simulink model "obs_based_state_xfer"  (Simulink 8.6)
settings: Solver=ode45  StartTime=0.0  StopTime=10.0  RelTol=1e-3
settings Model: Creator=Thomas Chmielewski  LastModifiedBy=DR_C
settings OptimizationCC: InitFltsAndDblsToZero=on
settings DebuggingCC: SaveWithParameterizedLinksMsg=none  SignalResolutionControl=TryResolveAllWithWarning  SolverPrmCheckMsg=none  MultiTaskDSMMsg=warning  MultiTaskCondExecSysMsg=none  FcnCallInpInsideContextMsg=UseLocalSettings  StrictBusMsg=None
settings HardwareCC: TargetUnknown=on
settings GRTTargetCC: TargetFcnLib=ansi_tfl_tmw.mat  CompOptLevelCompliant=off  GeneratePreprocessorConditionals=Use local settings

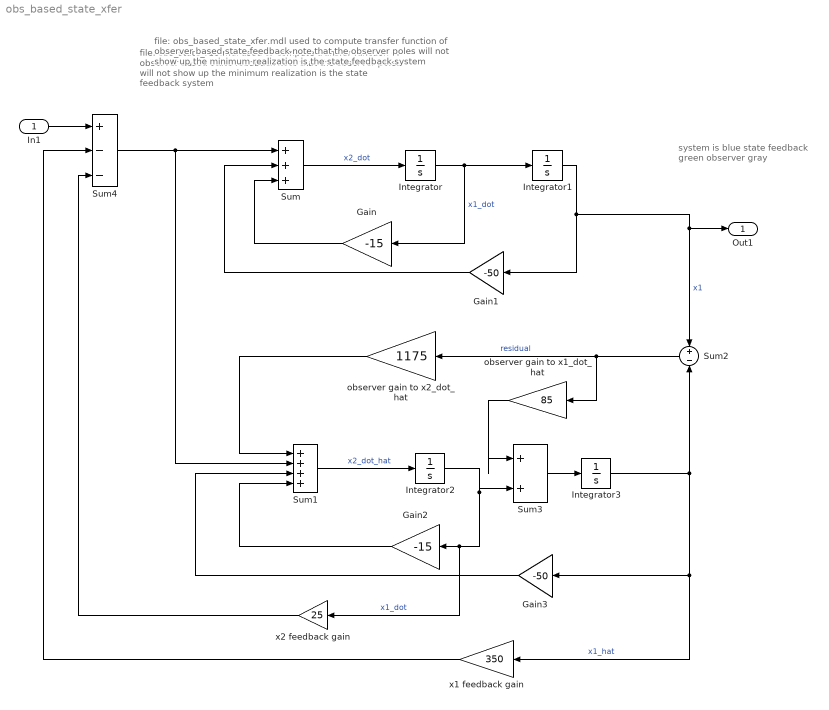
== system obs_based_state_xfer ==
  note: system is blue
      | state feedback green
      | observer gray
  note: file:  obs_state_r13.mdl
      | used to compute transfer function of
      | observer based state feedback
      | note that the observer poles will not show up
      | the minimum realization is the state feedback system
  note: file:  obs_based_state_xfer.mdl
      | used to compute transfer function of
      | observer based state feedback
      | note that the observer poles will not show up
      | the minimum realization is the state feedback system
  In1 : Inport
  Gain : Gain  Gain=-15
  Gain1 : Gain  Gain=-50
  Gain2 : Gain  Gain=-15
  Gain3 : Gain  Gain=-50
  Integrator{,1..3} (4 alike) : Integrator
  Sum : Sum  Inputs=+++
  Sum1 : Sum  Inputs=++++
  Sum2 : Sum  Inputs=+-
  Sum3 : Sum  Inputs=|++
  Sum4 : Sum  Inputs=+--
  observer gain to x1_dot_hat : Gain  Gain=85
  observer gain to x2_dot_hat : Gain  Gain=1175
  x1 feedback gain : Gain  Gain=350
  x2 feedback gain : Gain  Gain=25
  Out1 : Outport
  wires:
  Integrator/1 -> Integrator1/1, Gain/1  "x1_dot"
  Sum/1 -> Integrator/1  "x2_dot"
  Integrator1/1 -> Gain1/1, Sum2/1, Out1/1  "x1"
  Gain/1 -> Sum/3
  Gain1/1 -> Sum/2
  Integrator2/1 -> Sum3/2, Gain2/1, x2 feedback gain/1  "x1_dot"
  Sum1/1 -> Integrator2/1  "x2_dot_hat"
  Integrator3/1 -> Gain3/1, x1 feedback gain/1, Sum2/2  "x1_hat"
  Gain2/1 -> Sum1/4
  Gain3/1 -> Sum1/3
  observer gain to x2_dot_hat/1 -> Sum1/1
  Sum3/1 -> Integrator3/1
  observer gain to x1_dot_hat/1 -> Sum3/1
  Sum2/1 -> observer gain to x2_dot_hat/1, observer gain to x1_dot_hat/1  "residual"
  Sum4/1 -> Sum/1, Sum1/2
  x2 feedback gain/1 -> Sum4/3
  x1 feedback gain/1 -> Sum4/2
  In1/1 -> Sum4/1
